simulink model "CrC_VD"  (R2016b)
settings: configuration reference "CodeGenConfigSet" (kept outside this file)
values from neighbouring files (symbols this model uses):
  CrC_bCrCtlPrs_C = Calibration.Parameter    [init_CrC_VD.m]
  CrC_st3Btn_C = Calibration.Parameter    [init_CrC_VD.m]
undefined symbols (not defined in the file or in its folder): Switch_conv
libraries: simulink x18
settings Model: Creator=xinchangran  LastModifiedBy=xinchangran
settings ConfigSetRef: SourceLocation=Base Workspace

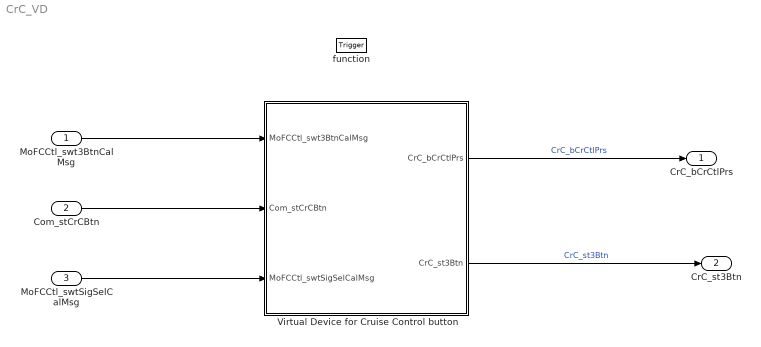
== system CrC_VD ==
  MoFCCtl_swt3BtnCalMsg : Inport  Description=digital inputs pins are used  OutMin=0  OutMax=255  OutDataTypeStr=State_uint8
  Com_stCrCBtn : Inport  Description=One source is CAN  Port=2  OutMin=0  OutMax=255  OutDataTypeStr=State_uint8
  MoFCCtl_swtSigSelCalMsg : Inport  Description=selection switch  Port=3  OutMin=0  OutMax=255  OutDataTypeStr=State_uint8
  function : TriggerPort  TriggerType=function-call  VariantControl=Variant
  Virtual Device for Cruise Control button : Subsystem
  CrC_bCrCtlPrs : Outport  Description=0：No cruise control unit present/1cruise control unit present  OutMin=0  OutMax=1  OutDataTypeStr=boolean
  CrC_st3Btn : Outport  Description=0：4 Button logic is used/1：3 Button logic is used  Port=2  OutMin=0  OutMax=1  OutDataTypeStr=boolean
  wires:
  MoFCCtl_swt3BtnCalMsg/1 -> Virtual Device for Cruise Control button/1(MoFCCtl_swt3BtnCalMsg)
  Com_stCrCBtn/1 -> Virtual Device for Cruise Control button/2(Com_stCrCBtn)
  MoFCCtl_swtSigSelCalMsg/1 -> Virtual Device for Cruise Control button/3(MoFCCtl_swtSigSelCalMsg)
  Virtual Device for Cruise Control button/1(CrC_bCrCtlPrs) -> CrC_bCrCtlPrs/1  "CrC_bCrCtlPrs"
  Virtual Device for Cruise Control button/2(CrC_st3Btn) -> CrC_st3Btn/1  "CrC_st3Btn"

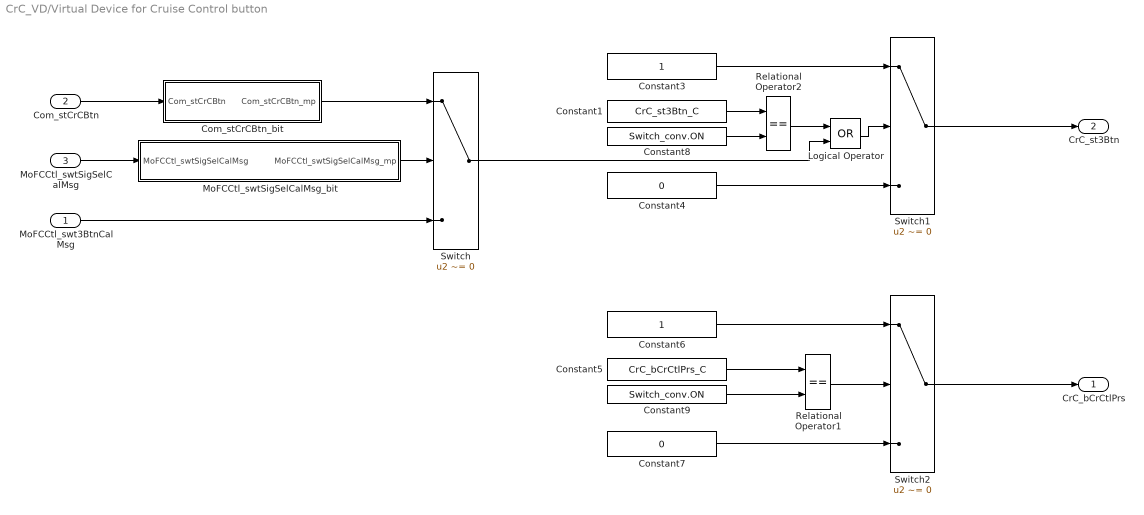
== system CrC_VD/Virtual Device for Cruise Control button ==
  MoFCCtl_swt3BtnCalMsg : Inport  Description=digital inputs pins are used  OutMin=0  OutMax=255  OutDataTypeStr=State_uint8
  Com_stCrCBtn : Inport  Description=One source is CAN  Port=2  OutMin=0  OutMax=255  OutDataTypeStr=State_uint8
  MoFCCtl_swtSigSelCalMsg : Inport  Description=selection switch  Port=3  OutMin=0  OutMax=255  OutDataTypeStr=State_uint8
  Com_stCrCBtn_bit : Subsystem
  Constant1 : Constant  Value=CrC_st3Btn_C
  Constant3 : Constant  OutDataTypeStr=Inherit: Inherit via back propagation
  Constant4 : Constant  Value=0  OutDataTypeStr=Inherit: Inherit via back propagation
  Constant5 : Constant  Value=CrC_bCrCtlPrs_C
  Constant6 : Constant  OutDataTypeStr=Inherit: Inherit via back propagation
  Constant7 : Constant  Value=0  OutDataTypeStr=Inherit: Inherit via back propagation
  Constant8 : Constant  Value=Switch_conv.ON
  Constant9 : Constant  Value=Switch_conv.ON
  Logical Operator : Logic  Operator=OR  AllPortsSameDT=off  OutDataTypeStr=boolean
  MoFCCtl_swtSigSelCalMsg_bit : Subsystem
  Relational Operator1 : RelationalOperator  Operator===  OutDataTypeStr=boolean  RndMeth=Nearest
  Relational Operator2 : RelationalOperator  Operator===  OutDataTypeStr=boolean  RndMeth=Nearest
  Switch : Switch  Criteria=u2 ~= 0  InputSameDT=on
  Switch1 : Switch  Criteria=u2 ~= 0  InputSameDT=on
  Switch2 : Switch  Criteria=u2 ~= 0  InputSameDT=on
  CrC_bCrCtlPrs : Outport  OutMin=0  OutMax=1  OutDataTypeStr=boolean
  CrC_st3Btn : Outport  Description=two sources for the 3/4 button logic information  Port=2  OutMin=0  OutMax=1  OutDataTypeStr=boolean
  wires:
  Com_stCrCBtn_bit/1(Com_stCrCBtn_mp) -> Switch/1
  Com_stCrCBtn/1 -> Com_stCrCBtn_bit/1(Com_stCrCBtn)
  MoFCCtl_swt3BtnCalMsg/1 -> Switch/3
  MoFCCtl_swtSigSelCalMsg/1 -> MoFCCtl_swtSigSelCalMsg_bit/1(MoFCCtl_swtSigSelCalMsg)
  MoFCCtl_swtSigSelCalMsg_bit/1(MoFCCtl_swtSigSelCalMsg_mp) -> Switch/2
  Constant4/1 -> Switch1/3
  Constant3/1 -> Switch1/1
  Switch2/1 -> CrC_bCrCtlPrs/1
  Constant1/1 -> Relational Operator2/1
  Constant8/1 -> Relational Operator2/2
  Switch1/1 -> CrC_st3Btn/1
  Constant7/1 -> Switch2/3
  Constant6/1 -> Switch2/1
  Relational Operator1/1 -> Switch2/2
  Constant5/1 -> Relational Operator1/1
  Constant9/1 -> Relational Operator1/2
  Switch/1 -> Logical Operator/2
  Relational Operator2/1 -> Logical Operator/1
  Logical Operator/1 -> Switch1/2

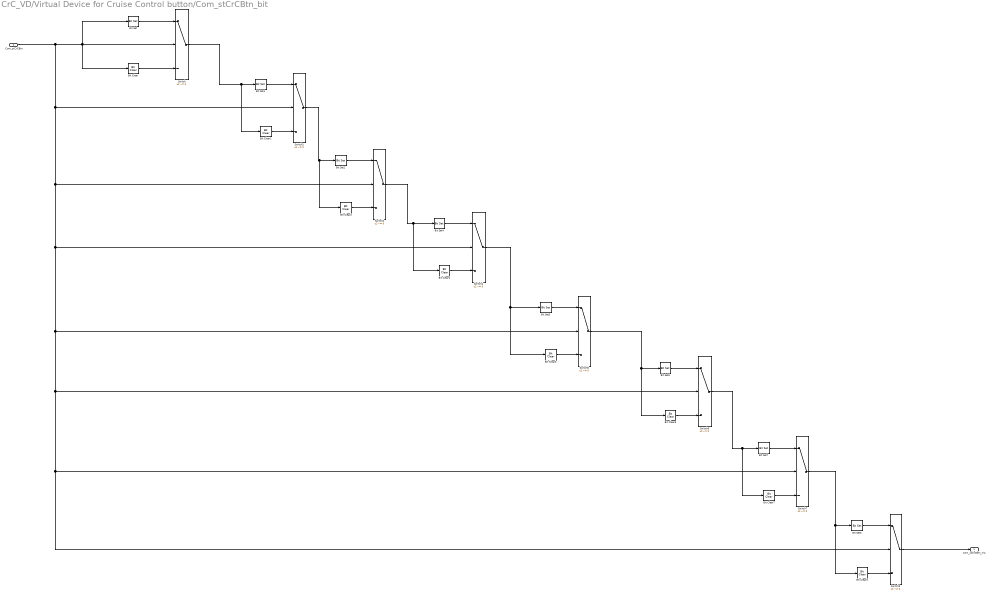
== system CrC_VD/Virtual Device for Cruise Control button/Com_stCrCBtn_bit ==
  Com_stCrCBtn : Inport
  Bit Clear : simulink/Logic and Bit Operations/Bit Clear  iBit=1
  Bit Clear1 : simulink/Logic and Bit Operations/Bit Clear  iBit=2
  Bit Clear2 : simulink/Logic and Bit Operations/Bit Clear  iBit=3
  Bit Clear3 : simulink/Logic and Bit Operations/Bit Clear  iBit=0
  Bit Clear4 : simulink/Logic and Bit Operations/Bit Clear  iBit=4
  Bit Clear5 : simulink/Logic and Bit Operations/Bit Clear  iBit=5
  Bit Clear6 : simulink/Logic and Bit Operations/Bit Clear  iBit=6
  Bit Clear7 : simulink/Logic and Bit Operations/Bit Clear  iBit=7
  Bit Set : simulink/Logic and Bit Operations/Bit Set  iBit=1
  Bit Set1 : simulink/Logic and Bit Operations/Bit Set  iBit=2
  Bit Set2 : simulink/Logic and Bit Operations/Bit Set  iBit=3
  Bit Set3 : simulink/Logic and Bit Operations/Bit Set  iBit=0
  Bit Set4 : simulink/Logic and Bit Operations/Bit Set  iBit=4
  Bit Set5 : simulink/Logic and Bit Operations/Bit Set  iBit=5
  Bit Set6 : simulink/Logic and Bit Operations/Bit Set  iBit=6
  Bit Set7 : simulink/Logic and Bit Operations/Bit Set  iBit=7
  Switch{,1..7} (8 alike) : Switch  Criteria=u2 ~= 0  InputSameDT=on
  Com_stCrCBtn_mp : Outport
  wires:
  Bit Clear6/1 -> Switch6/3
  Bit Set6/1 -> Switch6/1
  Bit Set3/1 -> Switch3/1
  Switch1/1 -> Bit Clear2/1, Bit Set2/1
  Bit Set2/1 -> Switch2/1
  Bit Clear3/1 -> Switch3/3
  Bit Clear2/1 -> Switch2/3
  Bit Set/1 -> Switch/1
  Bit Set1/1 -> Switch1/1
  Switch/1 -> Bit Clear1/1, Bit Set1/1
  Switch3/1 -> Com_stCrCBtn_mp/1
  Bit Clear1/1 -> Switch1/3
  Bit Clear/1 -> Switch/3
  Bit Clear5/1 -> Switch5/3
  Bit Set5/1 -> Switch5/1
  Bit Set4/1 -> Switch4/1
  Bit Clear4/1 -> Switch4/3
  Switch2/1 -> Bit Clear4/1, Bit Set4/1
  Bit Clear7/1 -> Switch7/3
  Bit Set7/1 -> Switch7/1
  Switch7/1 -> Bit Clear3/1, Bit Set3/1
  Switch5/1 -> Bit Clear6/1, Bit Set6/1
  Switch4/1 -> Bit Clear5/1, Bit Set5/1
  Switch6/1 -> Bit Clear7/1, Bit Set7/1
  Com_stCrCBtn/1 -> Switch6/2, Switch3/2, Switch7/2, Switch5/2, Switch4/2, Switch2/2, Switch1/2, Bit Clear/1, Bit Set/1, Switch/2

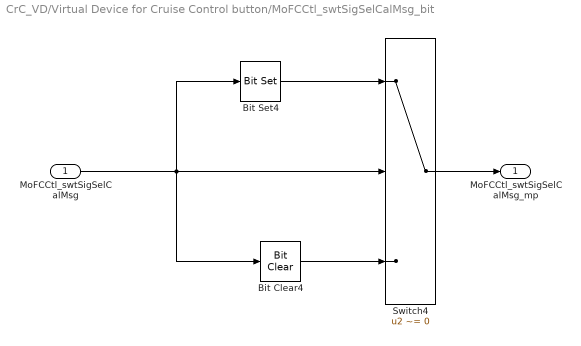
== system CrC_VD/Virtual Device for Cruise Control button/MoFCCtl_swtSigSelCalMsg_bit ==
  MoFCCtl_swtSigSelCalMsg : Inport
  Bit Clear4 : simulink/Logic and Bit Operations/Bit Clear  iBit=4
  Bit Set4 : simulink/Logic and Bit Operations/Bit Set  iBit=4
  Switch4 : Switch  Criteria=u2 ~= 0  InputSameDT=on
  MoFCCtl_swtSigSelCalMsg_mp : Outport
  wires:
  MoFCCtl_swtSigSelCalMsg/1 -> Switch4/2, Bit Set4/1, Bit Clear4/1
  Bit Clear4/1 -> Switch4/3
  Bit Set4/1 -> Switch4/1
  Switch4/1 -> MoFCCtl_swtSigSelCalMsg_mp/1
